simulink model "Controller_Designer"  (R2022a)
settings: Solver=VariableStepAuto  StartTime=0.0  StopTime=6  MaxStep=0.0001  RelTol=1e-3
undefined symbols (not defined in the file): DiscIntNeverNeededParam, MAX_I, P, REF_YAW_MAX, yaw_deadband, YAW_MAX
libraries: simulink x2
settings Model: FPTShortcutValueString='{{},{''BaselineRun_4'',1,1,1,''BaselineRun_4'','''',{},''M'',''D'',''''}}'  Creator=Inver  LastModifiedBy=Inver
settings DebuggingCC: SignalRangeChecking=warning

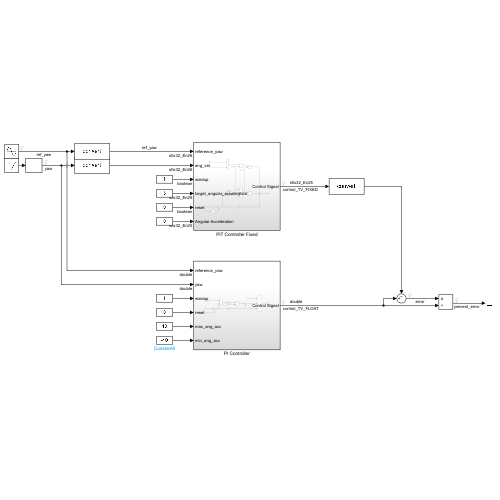
[thumbnail: Simulink's stored preview of the top-level diagram]
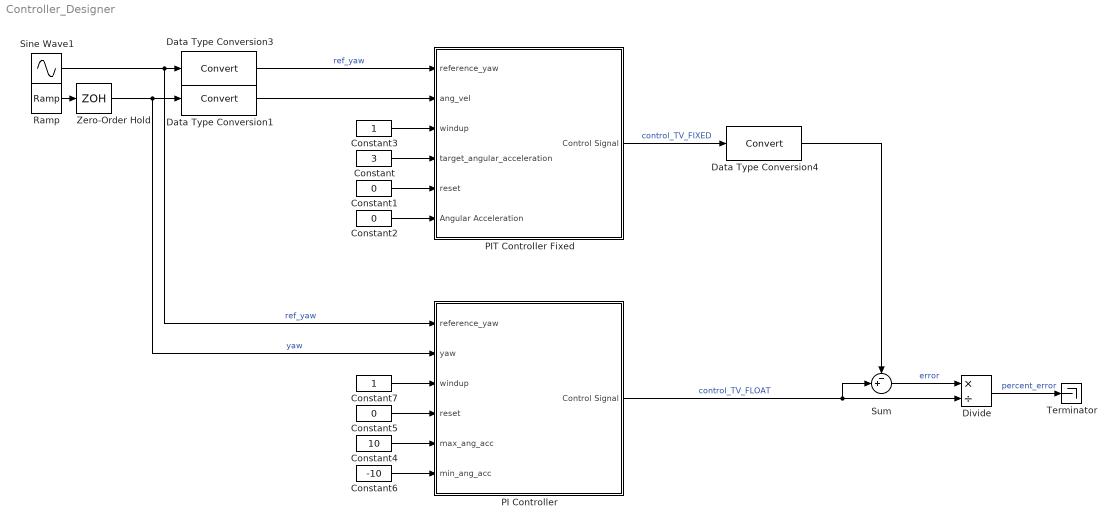
== system Controller_Designer ==
  Constant : Constant  Value=3  OutDataTypeStr=Inherit: Inherit via back propagation
  Constant1 : Constant  Value=0  OutDataTypeStr=boolean
  Constant2 : Constant  Value=0  OutDataTypeStr=Inherit: Inherit via back propagation
  Constant3 : Constant  OutDataTypeStr=boolean
  Constant4 : Constant  Value=10  OutDataTypeStr=boolean
  Constant5 : Constant  Value=0  OutDataTypeStr=boolean
  Constant6 : Constant  Value=-10  OutDataTypeStr=boolean
  Constant7 : Constant  OutDataTypeStr=boolean
  Data Type Conversion1 : DataTypeConversion  SaturateOnIntegerOverflow=off  RndMeth=Floor
  Data Type Conversion3 : DataTypeConversion  SaturateOnIntegerOverflow=off  RndMeth=Floor
  Data Type Conversion4 : DataTypeConversion  SaturateOnIntegerOverflow=off  RndMeth=Floor
  Divide : Product  Inputs=*/
  PI Controller : Subsystem
  PIT Controller Fixed : Subsystem
  Ramp : simulink/Sources/Ramp  slope=YAW_MAX  start=0  InitialOutput=0
  Sine Wave1 : Sin  Amplitude=REF_YAW_MAX  Frequency=2*pi  SampleTime=0
  Sum : Sum  Inputs=-+|
  Terminator : Terminator
  Zero-Order Hold : ZeroOrderHold
  wires:
  PIT Controller Fixed/1(Control Signal) -> Data Type Conversion4/1  "control_TV_FIXED"
  Zero-Order Hold/1 -> Data Type Conversion1/1, PI Controller/2(yaw)  "yaw"
  Sine Wave1/1 -> Data Type Conversion3/1, PI Controller/1(reference_yaw)  "ref_yaw"
  Data Type Conversion1/1 -> PIT Controller Fixed/2(ang_vel)
  PI Controller/1(Control Signal) -> Sum/2, Divide/2  "control_TV_FLOAT"
  Data Type Conversion3/1 -> PIT Controller Fixed/1(reference_yaw)  "ref_yaw"
  Data Type Conversion4/1 -> Sum/1
  Sum/1 -> Divide/1  "error"
  Divide/1 -> Terminator/1  "percent_error"
  Constant/1 -> PIT Controller Fixed/4(target_angular_acceleration)
  Constant2/1 -> PIT Controller Fixed/6(Angular Acceleration)
  Constant1/1 -> PIT Controller Fixed/5(reset)
  Constant3/1 -> PIT Controller Fixed/3(windup)
  Constant7/1 -> PI Controller/3(windup)
  Constant5/1 -> PI Controller/4(reset)
  Ramp/1 -> Zero-Order Hold/1
  Constant4/1 -> PI Controller/5(max_ang_acc)
  Constant6/1 -> PI Controller/6(min_ang_acc)

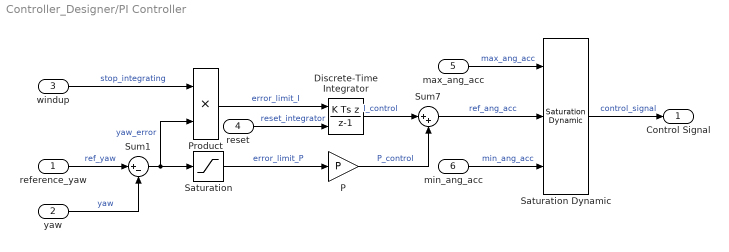
== system Controller_Designer/PI Controller ==
  reference_yaw : Inport  OutDataTypeStr=double  LockScale=on
  yaw : Inport  Port=2  OutDataTypeStr=double  LockScale=on
  windup : Inport  Port=3  PortDimensions=1  LockScale=on
  reset : Inport  Port=4  LockScale=on
  max_ang_acc : Inport  Port=5  PortDimensions=1  LockScale=on
  min_ang_acc : Inport  Port=6  PortDimensions=1  LockScale=on
  Discrete-Time Integrator : DiscreteIntegrator  IntegratorMethod=Integration: Backward Euler  gainval=I  ExternalReset=level  SampleTime=-1  OutDataTypeStr=Inherit: Inherit via back propagation  LimitOutput=on  UpperSaturationLimit=MAX_I  LowerSaturationLimit=-MAX_I  ICPrevOutput=DiscIntNeverNeededParam  ICPrevScaledInput=DiscIntNeverNeededParam
  P : Gain  Gain=P  ParamDataTypeStr=double  OutDataTypeStr=double
  Product : Product
  Saturation : Saturate  UpperLimit=YAW_MAX  LowerLimit=-YAW_MAX
  Saturation Dynamic : simulink/Discontinuities/Saturation Dynamic  OutMin=[]  OutMax=[]  OutDataTypeStr=Inherit: Same as second input  OutDataType=fixdt(1, 16)  OutScaling=2^-10  DoSatur=off
  Sum1 : Sum  Inputs=|+-  OutDataTypeStr=Inherit: Inherit via back propagation
  Sum7 : Sum  Inputs=|++  OutDataTypeStr=double  SaturateOnIntegerOverflow=on
  Control Signal : Outport  OutDataTypeStr=double  PortDimensions=1  LockScale=on
  wires:
  P/1 -> Sum7/2  "P_control"
  windup/1 -> Product/1  "stop_integrating"
  Sum1/1 -> Saturation/1, Product/2  "yaw_error"
  reset/1 -> Discrete-Time Integrator/2  "reset_integrator"
  yaw/1 -> Sum1/2  "yaw"
  Discrete-Time Integrator/1 -> Sum7/1  "I_control"
  reference_yaw/1 -> Sum1/1  "ref_yaw"
  Product/1 -> Discrete-Time Integrator/1  "error_limit_I"
  Sum7/1 -> Saturation Dynamic/2  "ref_ang_acc"
  Saturation Dynamic/1 -> Control Signal/1  "control_signal"
  max_ang_acc/1 -> Saturation Dynamic/1  "max_ang_acc"
  min_ang_acc/1 -> Saturation Dynamic/3  "min_ang_acc"
  Saturation/1 -> P/1  "error_limit_P"

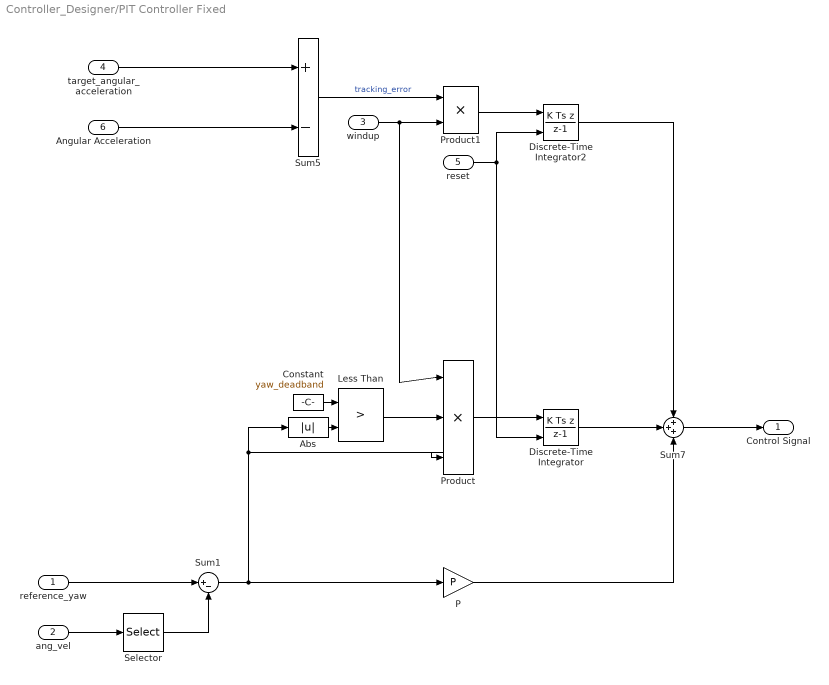
== system Controller_Designer/PIT Controller Fixed ==
  reference_yaw : Inport  OutDataTypeStr=fixdt(1,32,26)  LockScale=on
  ang_vel : Inport  Port=2  OutDataTypeStr=fixdt(1,32,26)  LockScale=on
  windup : Inport  Port=3  OutDataTypeStr=boolean  LockScale=on
  target_angular_acceleration : Inport  Port=4  OutDataTypeStr=fixdt(1,32,25)  LockScale=on
  reset : Inport  Port=5  OutDataTypeStr=boolean  LockScale=on
  Angular Acceleration : Inport  Port=6  OutDataTypeStr=fixdt(1,32,25)  LockScale=on
  Abs : Abs  OutDataTypeStr=Inherit: Inherit via back propagation  SaturateOnIntegerOverflow=off
  Constant : Constant  Value=yaw_deadband  OutDataTypeStr=fixdt(0,16,15)
  Discrete-Time Integrator : DiscreteIntegrator  IntegratorMethod=Integration: Backward Euler  gainval=I  ExternalReset=level  SampleTime=-1  OutDataTypeStr=Inherit: Inherit via back propagation  LimitOutput=on  UpperSaturationLimit=10  LowerSaturationLimit=-10  ICPrevOutput=DiscIntNeverNeededParam  ICPrevScaledInput=DiscIntNeverNeededParam
  Discrete-Time Integrator2 : DiscreteIntegrator  IntegratorMethod=Integration: Backward Euler  gainval=T  ExternalReset=level  SampleTime=-1  OutDataTypeStr=Inherit: Inherit via back propagation  LimitOutput=on  UpperSaturationLimit=10  LowerSaturationLimit=-10  ICPrevOutput=DiscIntNeverNeededParam  ICPrevScaledInput=DiscIntNeverNeededParam
  Less Than : RelationalOperator  Operator=>  OutDataTypeStr=boolean  RndMeth=Simplest  InputSameDT=off
  P : Gain  Gain=P  ParamDataTypeStr=double  OutDataTypeStr=fixdt(1,32,25)
  Product : Product  Inputs=3  OutDataTypeStr=Inherit: Inherit via back propagation
  Product1 : Product  OutDataTypeStr=Inherit: Inherit via back propagation
  Selector : Selector  InputPortWidth=3  IndexOptions=Index vector (dialog)  Indices=3  OutputSizes=1
  Sum1 : Sum  Inputs=|+-  OutDataTypeStr=Inherit: Inherit via back propagation
  Sum5 : Sum  Inputs=+-  OutDataTypeStr=Inherit: Same as accumulator
  Sum7 : Sum  Inputs=+++  OutDataTypeStr=Inherit: Inherit via back propagation  SaturateOnIntegerOverflow=on
  Control Signal : Outport  OutDataTypeStr=fixdt(1,32,25)  LockScale=on
  wires:
  Sum5/1 -> Product1/1  "tracking_error"
  P/1 -> Sum7/3
  windup/1 -> Product/1, Product1/2
  Product/1 -> Discrete-Time Integrator/1
  Sum1/1 -> Abs/1, Product/3, P/1
  target_angular_acceleration/1 -> Sum5/1
  Angular Acceleration/1 -> Sum5/2
  Product1/1 -> Discrete-Time Integrator2/1
  reset/1 -> Discrete-Time Integrator2/2, Discrete-Time Integrator/2
  Abs/1 -> Less Than/2
  Constant/1 -> Less Than/1
  Less Than/1 -> Product/2
  Selector/1 -> Sum1/2
  Sum7/1 -> Control Signal/1
  ang_vel/1 -> Selector/1
  Discrete-Time Integrator2/1 -> Sum7/1
  Discrete-Time Integrator/1 -> Sum7/2
  reference_yaw/1 -> Sum1/1
